simulink model "LQR_dis_red"  (R2023b)
settings: Solver=VariableStepAuto  StartTime=0.0  StopTime=200  RelTol=1e-3
undefined symbols (not defined in the file): A_red, B_total_red, C_ss_red, CI_red, DI_red, DiscIntNeverNeededParam, dVdt, K_red, Kint_red, ramp_wd, step_temp, steptime, Ts, Tsp_red, Ufeedforward_red, V0, Vb0, Vmax, Vmin
libraries: simulink x2
settings Model: Creator=Maialen  LastModifiedBy=Maialen

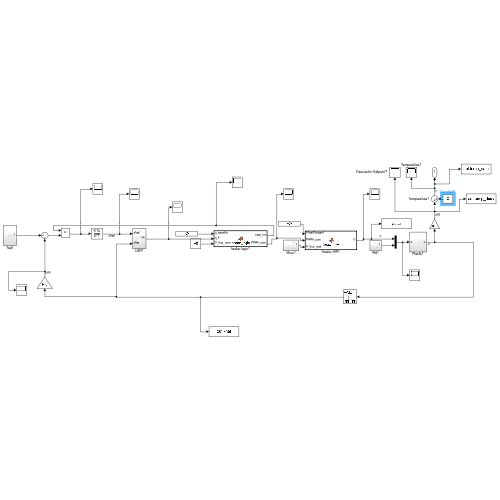
[thumbnail: Simulink's stored preview of the top-level diagram]
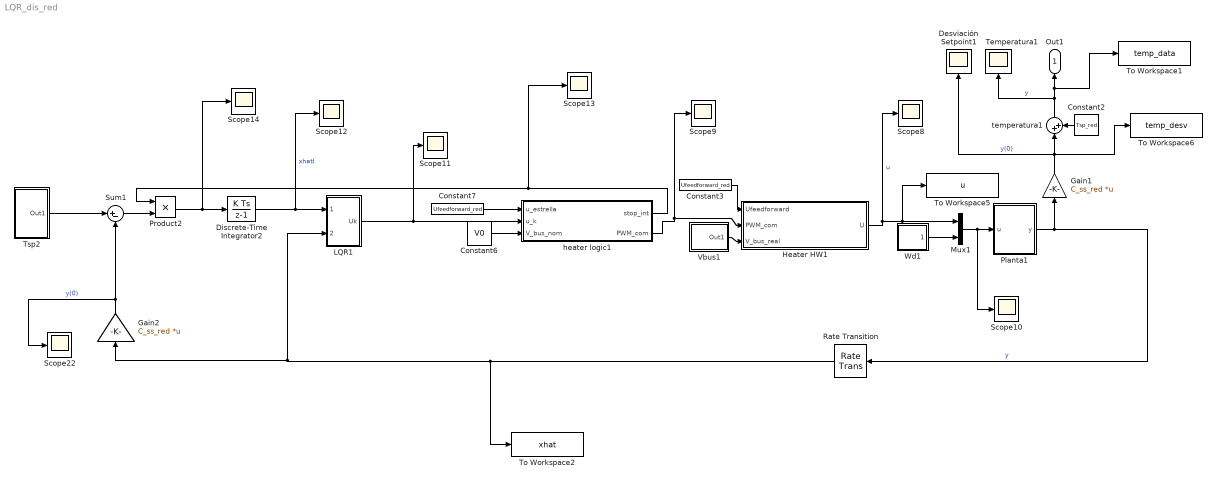
== system LQR_dis_red ==
  Constant2 : Constant  Value=Tsp_red  SampleTime=0
  Constant3 : Constant  Value=Ufeedforward_red  SampleTime=0
  Constant6 : Constant  Value=V0  SampleTime=0
  Constant7 : Constant  Value=Ufeedforward_red  SampleTime=0
  Desviación Setpoint1 : Scope
  Discrete-Time Integrator2 : DiscreteIntegrator  SampleTime=Ts  ICPrevOutput=DiscIntNeverNeededParam  ICPrevScaledInput=DiscIntNeverNeededParam
  Gain1 : Gain  Gain=C_ss_red  Multiplication=Matrix(K*u)
  Gain2 : Gain  Gain=C_ss_red  Multiplication=Matrix(K*u)
  Heater HW1 : MATLAB Function  TreatAsAtomicUnit=on
  LQR1 : Subsystem
  Mux1 : Mux  Inputs=2
  Planta1 : Subsystem
  Product2 : Product
  Rate Transition : RateTransition  OutPortSampleTime=Ts
  Scope{8..14,22} (8 alike) : Scope
  Sum1 : Sum  Inputs=|+-
  Temperatura1 : Scope
  To Workspace1 : ToWorkspace  VariableName=temp_data  SaveFormat=Timeseries  SampleTime=-1
  To Workspace2 : ToWorkspace  VariableName=xhat  SaveFormat=Timeseries  SampleTime=-1
  To Workspace5 : ToWorkspace  VariableName=u  SaveFormat=Timeseries  SampleTime=-1
  To Workspace6 : ToWorkspace  VariableName=temp_desv  SaveFormat=Timeseries  SampleTime=-1
  Tsp2 : Subsystem
  Vbus1 : Subsystem
  Wd1 : Subsystem
  heater logic1 : MATLAB Function  TreatAsAtomicUnit=on
  temperatura1 : Sum  Inputs=|++
  Out1 : Outport
  wires:
  Constant6/1 -> heater logic1/3(V_bus_nom)
  Gain1/1 -> temperatura1/1, To Workspace6/1, Desviación Setpoint1/1  "y(0)"
  Product2/1 -> Discrete-Time Integrator2/1, Scope14/1
  Gain2/1 -> Sum1/2, Scope22/1  "y(0)"
  Constant3/1 -> Heater HW1/1(Ufeedforward)
  Discrete-Time Integrator2/1 -> Scope12/1, LQR1/1(xhatI)  "xhatI"
  Mux1/1 -> Scope10/1, Planta1/1(u)
  Heater HW1/1(U) -> To Workspace5/1, Mux1/1, Scope8/1  "u"
  heater logic1/1(stop_int) -> Scope13/1, Product2/1
  Constant7/1 -> heater logic1/1(u_estrella)
  LQR1/1(Uk) -> Scope11/1, heater logic1/2(u_k)
  Wd1/1(Out1) -> Mux1/2
  Sum1/1 -> Product2/2
  heater logic1/2(PWM_com) -> Heater HW1/2(PWM_com), Scope9/1
  temperatura1/1 -> Temperatura1/1, To Workspace1/1, Out1/1  "y"
  Planta1/1(y) -> Rate Transition/1, Gain1/1  "y"
  Constant2/1 -> temperatura1/2
  Tsp2/1(Out1) -> Sum1/1
  Rate Transition/1 -> To Workspace2/1, LQR1/2(xhat), Gain2/1
  Vbus1/1(Out1) -> Heater HW1/3(V_bus_real)

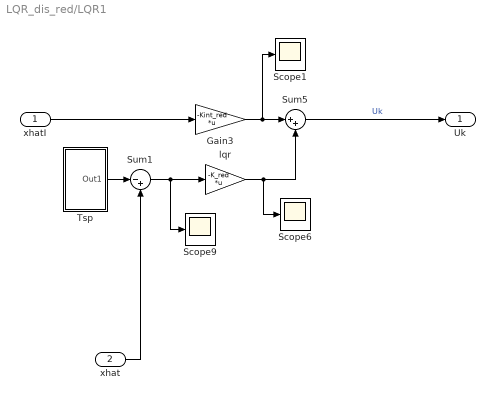
== system LQR_dis_red/LQR1 ==
  xhatI : Inport
  xhat : Inport  Port=2
  Gain3 : Gain  Gain=-Kint_red  Multiplication=Matrix(K*u)
  Scope1 : Scope
  Scope6 : Scope
  Scope9 : Scope
  Sum1 : Sum  Inputs=|-+
  Sum5 : Sum  Inputs=|++
  Tsp : Subsystem
  lqr : Gain  Gain=-K_red  Multiplication=Matrix(K*u)
  Uk : Outport
  wires:
  xhatI/1 -> Gain3/1
  Sum5/1 -> Uk/1  "Uk"
  lqr/1 -> Scope6/1, Sum5/2
  Gain3/1 -> Scope1/1, Sum5/1
  Sum1/1 -> Scope9/1, lqr/1
  Tsp/1(Out1) -> Sum1/1
  xhat/1 -> Sum1/2

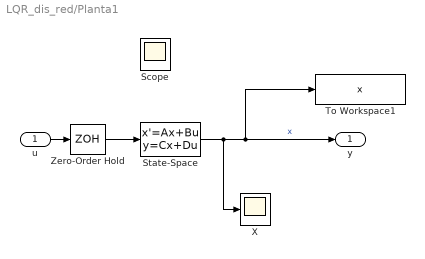
== system LQR_dis_red/Planta1 ==
  u : Inport
  Scope : Scope
  State-Space : StateSpace  A=A_red  B=B_total_red  C=CI_red  D=DI_red  InitialCondition=0
  To Workspace1 : ToWorkspace  VariableName=x  SaveFormat=Timeseries  SampleTime=-1
  X : Scope
  Zero-Order Hold : ZeroOrderHold  SampleTime=Ts
  y : Outport
  wires:
  State-Space/1 -> To Workspace1/1, y/1, X/1  "x"
  u/1 -> Zero-Order Hold/1
  Zero-Order Hold/1 -> State-Space/1

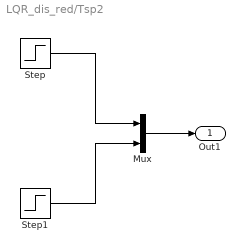
== system LQR_dis_red/Tsp2 ==
  Mux : Mux  Inputs=2
  Step : Step  Time=steptime  After=step_temp  SampleTime=0
  Step1 : Step  Time=steptime  After=step_temp  SampleTime=0
  Out1 : Outport
  wires:
  Mux/1 -> Out1/1
  Step/1 -> Mux/1
  Step1/1 -> Mux/2

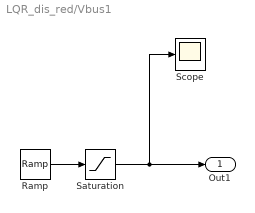
== system LQR_dis_red/Vbus1 ==
  Ramp : simulink/Sources/Ramp  slope=dVdt  start=steptime  InitialOutput=Vb0
  Saturation : Saturate  UpperLimit=Vmax  LowerLimit=Vmin
  Scope : Scope
  Out1 : Outport
  wires:
  Ramp/1 -> Saturation/1
  Saturation/1 -> Scope/1, Out1/1

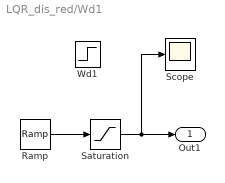
== system LQR_dis_red/Wd1 ==
  Ramp : simulink/Sources/Ramp  slope=ramp_wd  start=steptime  InitialOutput=0
  Saturation : Saturate  LowerLimit=-1
  Scope : Scope
  Wd1 : Step  Time=steptime  After=0  SampleTime=0
  Out1 : Outport
  wires:
  Ramp/1 -> Saturation/1
  Saturation/1 -> Scope/1, Out1/1

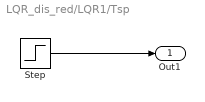
== system LQR_dis_red/LQR1/Tsp ==
  Step : Step  Time=steptime  After=step_temp  SampleTime=0
  Out1 : Outport
  wires:
  Step/1 -> Out1/1

== matlab function LQR_dis_red/Heater HW1 ==
  data: Ufeedforward input; PWM_com input; U output; V_bus_real input
function U = heater_hw(Ufeedforward, PWM_com, V_bus_real)
    R_real = [156.8; 156.8];

    % Potencia real entregada a la planta
    P_max_real = (V_bus_real^2) ./ R_real;
    U = PWM_com .* P_max_real - Ufeedforward;
end
% 
% function U = heater_hw(u_estrella, PWM_com, V_bus_real)
%     R_real = [135.2; 135.2];
%     P_max_real = (V_bus_real^2) ./ R_real;
%     P_entregada = PWM_com .* P_max_real;
%     P_entregada = max(0, P_entregada);  % protección física
%     U = P_entregada - u_estrella;
% end

== matlab function LQR_dis_red/heater logic1 ==
  data: stop_int output; u_estrella input; u_k input; PWM_com output; V_bus_nom input
function [stop_int, PWM_com] = heater_logic(u_estrella, u_k, V_bus_nom)
    R0 = [156.8; 156.8];
    
    % Potencia máxima disponible
    P_max = (V_bus_nom^2) ./ R0;
    
    % Potencia absoluta demandada = feedforward + corrección LQR (desviación)
    P_demanda =  u_k + u_estrella;
    
    % Saturación física
    P_limitada = max(0, min(P_max, P_demanda));
    
    % PWM lineal
    PWM_com = P_limitada ./ P_max;
    
    % Anti-windup: congela integrador si satura
    sat_arriba = P_demanda >= P_max;
    sat_abajo  = P_demanda <= 0;
    stop_int   = double(~(sat_arriba | sat_abajo));
   
end
